simulink model "pd_path_sg"  (R2013b)
settings: Solver=ode45  StartTime=0.0  StopTime=10  RelTol=1e-3
undefined symbols (not defined in the file or in its folder): A, A2, B, C, D, EVAL, i, output_samp_bcoef, PCIN, reg_pk_lim, reg_plim, reg_scale, reg_sr_lim, reg_staclr, reg_txgain, THIS_DATE, W, X, Z
undefined symbols (not defined in the file): lut_address, lut_address_s5, reg_dltap
libraries: xbsIndex_r4 x3819, lut_ram_vhdl x32
(part 11 of 31)

== system pd_path_sg/output_sw_B/add_switch ==
  chi : Inport
  x : Inport  Port=2
  d : Inport  Port=3
  on0 : Inport  Port=4
  on1 : Inport  Port=5
  AddSub1 : xbsIndex_r4/AddSub  mode=Addition  use_carryin=off  use_carryout=off  en=off  latency=1  precision=User Defined  arith_type="Signed  (2's comp)"  n_bits=17  bin_pt=0  quantization=Truncate  overflow=Wrap  use_behavioral_HDL=off  hw_selection=Fabric  pipelined=off  dbl_ovrd=off  block_type=addsub
  AddSub2 : xbsIndex_r4/AddSub  mode=Addition  use_carryin=off  use_carryout=off  en=off  latency=1  precision=User Defined  arith_type="Signed  (2's comp)"  n_bits=17  bin_pt=0  quantization=Truncate  overflow=Wrap  use_behavioral_HDL=off  hw_selection=Fabric  pipelined=off  dbl_ovrd=off  block_type=addsub
  Constant : xbsIndex_r4/Constant  const=0  gui_display_data_type=Fixed-point  arith_type=Signed (2's comp)  n_bits=17  bin_pt=0  preci_type=Single  exp_width=8  frac_width=24  explicit_period=off  period=1  equ=P=C  opselect=C  inp2=PCIN>>17  opr=+  inp1=P  carry=CIN  dbl_ovrd=off  block_type=constant
  Constant1 : xbsIndex_r4/Constant  const=0  gui_display_data_type=Fixed-point  arith_type=Signed (2's comp)  n_bits=17  bin_pt=0  preci_type=Single  exp_width=8  frac_width=24  explicit_period=off  period=1  equ=P=C  opselect=C  inp2=PCIN>>17  opr=+  inp1=P  carry=CIN  dbl_ovrd=off  block_type=constant
  Delay : xbsIndex_r4/Delay  rst=off  infoeditControl=Selection of Reset will increase slice count due to use of real FFs and instead of SRLs  en=off  latency=delaytaps+1  reg_retiming=off  dbl_ovrd=off  block_type=delay
      settings: infoedit=Hardware notes: A delay line is a chain, each link of which is an SRL16 or SRL32 followed by a flip-flop.
  Delay1 : xbsIndex_r4/Delay  rst=off  infoeditControl=Selection of Reset will increase slice count due to use of real FFs and instead of SRLs  en=off  latency=delaytaps+1  reg_retiming=off  dbl_ovrd=off  block_type=delay
      settings: infoedit=Hardware notes: A delay line is a chain, each link of which is an SRL16 or SRL32 followed by a flip-flop.
  Delay2 : xbsIndex_r4/Delay  rst=off  infoeditControl=Selection of Reset will increase slice count due to use of real FFs and instead of SRLs  en=off  latency=delaytaps  reg_retiming=off  dbl_ovrd=off  block_type=delay
      settings: infoedit=Hardware notes: A delay line is a chain, each link of which is an SRL16 or SRL32 followed by a flip-flop.
  Delay3 : xbsIndex_r4/Delay  rst=off  infoeditControl=Selection of Reset will increase slice count due to use of real FFs and instead of SRLs  en=off  latency=delaytaps  reg_retiming=off  dbl_ovrd=off  block_type=delay
      settings: infoedit=Hardware notes: A delay line is a chain, each link of which is an SRL16 or SRL32 followed by a flip-flop.
  Delay4 : xbsIndex_r4/Delay  rst=off  infoeditControl=Selection of Reset will increase slice count due to use of real FFs and instead of SRLs  en=off  latency=delaytaps  reg_retiming=off  dbl_ovrd=off  block_type=delay
      settings: infoedit=Hardware notes: A delay line is a chain, each link of which is an SRL16 or SRL32 followed by a flip-flop.
  Delay5 : xbsIndex_r4/Delay  rst=off  infoeditControl=Selection of Reset will increase slice count due to use of real FFs and instead of SRLs  en=off  latency=2  reg_retiming=off  dbl_ovrd=off  block_type=delay
      settings: infoedit=Hardware notes: A delay line is a chain, each link of which is an SRL16 or SRL32 followed by a flip-flop.
  Demux1 : Demux  Outputs=2
  Demux2 : Demux  Outputs=2
  Mux : xbsIndex_r4/Mux  inputs=2  en=off  latency=1  precision=Full  arith_type=Unsigned  n_bits=16  bin_pt=14  quantization=Truncate  overflow=Wrap  dbl_ovrd=off  block_type=mux
  Mux1 : xbsIndex_r4/Mux  inputs=2  en=off  latency=0  precision=Full  arith_type=Unsigned  n_bits=16  bin_pt=14  quantization=Truncate  overflow=Wrap  dbl_ovrd=off  block_type=mux
  Mux2 : xbsIndex_r4/Mux  inputs=2  en=off  latency=1  precision=Full  arith_type=Unsigned  n_bits=16  bin_pt=14  quantization=Truncate  overflow=Wrap  dbl_ovrd=off  block_type=mux
  Mux3 : Mux  Inputs=2
  cho : Outport
  y : Outport  Port=2
  wires:
  Mux1/1 -> Mux/1, Mux2/1
  Delay5/1 -> cho/1
  Delay4/1 -> Mux1/1, Delay5/1
  Delay3/1 -> Mux2/3
  Delay2/1 -> Mux/3
  Delay1/1 -> AddSub2/1
  Delay/1 -> AddSub1/1
  Mux3/1 -> y/1
  AddSub2/1 -> Mux3/2
  AddSub1/1 -> Mux3/1
  Mux2/1 -> AddSub2/2
  Mux/1 -> AddSub1/2
  Demux2/2 -> Delay3/1
  Demux2/1 -> Delay2/1
  Constant1/1 -> Mux2/2
  Demux1/2 -> Delay1/1
  Demux1/1 -> Delay/1
  d/1 -> Demux2/1
  x/1 -> Demux1/1
  chi/1 -> Delay4/1
  on1/1 -> Mux1/3
  on0/1 -> Mux1/2
  Constant/1 -> Mux/2

== system pd_path_sg/output_sw_B/ch_split ==
  per : Inport
  chnsel : Inport  Port=2
  Bus Creator : BusCreator  Inputs=3
  Bus Creator1 : BusCreator  Inputs=3
  Bus Selector : BusSelector  OutputSignals=addr,din,we
  Constant : xbsIndex_r4/Constant  const=0  gui_display_data_type=Boolean  arith_type=Boolean  n_bits=16  bin_pt=14  preci_type=Single  exp_width=8  frac_width=24  explicit_period=off  period=1  equ=P=C  opselect=C  inp2=PCIN>>17  opr=+  inp1=P  carry=CIN  dbl_ovrd=off  block_type=constant
  Constant1 : xbsIndex_r4/Constant  const=0  gui_display_data_type=Boolean  arith_type=Boolean  n_bits=16  bin_pt=14  preci_type=Single  exp_width=8  frac_width=24  explicit_period=off  period=1  equ=P=C  opselect=C  inp2=PCIN>>17  opr=+  inp1=P  carry=CIN  dbl_ovrd=off  block_type=constant
  Mux : xbsIndex_r4/Mux  inputs=2  en=off  latency=0  precision=Full  arith_type=Unsigned  n_bits=16  bin_pt=14  quantization=Truncate  overflow=Wrap  dbl_ovrd=off  block_type=mux
  Mux1 : xbsIndex_r4/Mux  inputs=2  en=off  latency=0  precision=Full  arith_type=Unsigned  n_bits=16  bin_pt=14  quantization=Truncate  overflow=Wrap  dbl_ovrd=off  block_type=mux
  per0 : Outport
  per1 : Outport  Port=2
  wires:
  Bus Creator/1 -> per0/1
  Mux/1 -> Bus Creator/3  "we"
  Bus Creator1/1 -> per1/1
  Mux1/1 -> Bus Creator1/3  "we"
  Constant1/1 -> Mux1/2
  Bus Selector/3 -> Mux/2, Mux1/3  "<we>"
  Constant/1 -> Mux/3
  chnsel/1 -> Mux/1, Mux1/1
  Bus Selector/2 -> Bus Creator/2, Bus Creator1/2  "<din>"
  Bus Selector/1 -> Bus Creator/1, Bus Creator1/1  "<addr>"
  per/1 -> Bus Selector/1

== system pd_path_sg/output_sw_B/config_regs0 ==
  per : Inport
  rst : Inport  Port=2
  B0 : xbsIndex_r4/Slice  nbits=1  boolean_output=on  mode=Lower Bit Location + Width  bit1=0  base1=MSB of Input  bit0=0  base0=LSB of Input  dbl_ovrd=off  block_type=slice
  B1 : xbsIndex_r4/Slice  nbits=1  boolean_output=on  mode=Lower Bit Location + Width  bit1=0  base1=MSB of Input  bit0=1  base0=LSB of Input  dbl_ovrd=off  block_type=slice
  B2 : xbsIndex_r4/Slice  nbits=16  boolean_output=off  mode=Lower Bit Location + Width  bit1=0  base1=MSB of Input  bit0=0  base0=LSB of Input  dbl_ovrd=off  block_type=slice
  Bus Selector : BusSelector  OutputSignals=addr,din,we
  Slice : xbsIndex_r4/Slice  nbits=16  boolean_output=off  mode=Lower Bit Location + Width  bit1=0  base1=MSB of Input  bit0=0  base0=LSB of Input  dbl_ovrd=off  block_type=slice
  Slice1 : xbsIndex_r4/Slice  nbits=16  boolean_output=off  mode=Lower Bit Location + Width  bit1=0  base1=MSB of Input  bit0=0  base0=LSB of Input  dbl_ovrd=off  block_type=slice
  perbus_reg : Subsystem
  perbus_reg1 : Subsystem
  perbus_reg2 : Subsystem
  perbus_reg3 : Subsystem
  sr_lim : Outport
  pk_lim : Outport  Port=2
  alarm_clr : Outport  Port=3
  pd_on : Outport  Port=4
  tx_gain : Outport  Port=5
  wires:
  rst/1 -> perbus_reg3/4(rst), perbus_reg2/4(rst)
  B2/1 -> tx_gain/1
  perbus_reg3/1(q) -> B2/1
  B1/1 -> pd_on/1
  B0/1 -> alarm_clr/1
  perbus_reg2/1(q) -> B0/1, B1/1
  per/1 -> Bus Selector/1
  Bus Selector/1 -> perbus_reg/1(addr), perbus_reg1/1(addr), perbus_reg2/1(addr), perbus_reg3/1(addr)  "<addr>"
  Bus Selector/2 -> perbus_reg/2(din), perbus_reg2/2(din), perbus_reg3/2(din), perbus_reg1/2(din)  "<din>"
  Bus Selector/3 -> perbus_reg/3(we), perbus_reg1/3(we), perbus_reg2/3(we), perbus_reg3/3(we)  "<we>"
  perbus_reg/1(q) -> Slice/1
  perbus_reg1/1(q) -> Slice1/1
  Slice/1 -> sr_lim/1
  Slice1/1 -> pk_lim/1

== system pd_path_sg/output_sw_B/config_regs1 ==
  per : Inport
  rst : Inport  Port=2
  B0 : xbsIndex_r4/Slice  nbits=1  boolean_output=on  mode=Lower Bit Location + Width  bit1=0  base1=MSB of Input  bit0=0  base0=LSB of Input  dbl_ovrd=off  block_type=slice
  B1 : xbsIndex_r4/Slice  nbits=1  boolean_output=on  mode=Lower Bit Location + Width  bit1=0  base1=MSB of Input  bit0=1  base0=LSB of Input  dbl_ovrd=off  block_type=slice
  B2 : xbsIndex_r4/Slice  nbits=16  boolean_output=off  mode=Lower Bit Location + Width  bit1=0  base1=MSB of Input  bit0=0  base0=LSB of Input  dbl_ovrd=off  block_type=slice
  Bus Selector : BusSelector  OutputSignals=addr,din,we
  Slice : xbsIndex_r4/Slice  nbits=16  boolean_output=off  mode=Lower Bit Location + Width  bit1=0  base1=MSB of Input  bit0=0  base0=LSB of Input  dbl_ovrd=off  block_type=slice
  Slice1 : xbsIndex_r4/Slice  nbits=16  boolean_output=off  mode=Lower Bit Location + Width  bit1=0  base1=MSB of Input  bit0=0  base0=LSB of Input  dbl_ovrd=off  block_type=slice
  perbus_reg : Subsystem
  perbus_reg1 : Subsystem
  perbus_reg2 : Subsystem
  perbus_reg3 : Subsystem
  sr_lim : Outport
  pk_lim : Outport  Port=2
  alarm_clr : Outport  Port=3
  pd_on : Outport  Port=4
  tx_gain : Outport  Port=5
  wires:
  Slice1/1 -> pk_lim/1
  Slice/1 -> sr_lim/1
  perbus_reg1/1(q) -> Slice1/1
  perbus_reg/1(q) -> Slice/1
  Bus Selector/3 -> perbus_reg3/3(we), perbus_reg2/3(we), perbus_reg1/3(we), perbus_reg/3(we)  "<we>"
  Bus Selector/2 -> perbus_reg1/2(din), perbus_reg3/2(din), perbus_reg2/2(din), perbus_reg/2(din)  "<din>"
  Bus Selector/1 -> perbus_reg3/1(addr), perbus_reg2/1(addr), perbus_reg1/1(addr), perbus_reg/1(addr)  "<addr>"
  per/1 -> Bus Selector/1
  perbus_reg2/1(q) -> B1/1, B0/1
  B0/1 -> alarm_clr/1
  B1/1 -> pd_on/1
  perbus_reg3/1(q) -> B2/1
  B2/1 -> tx_gain/1
  rst/1 -> perbus_reg2/4(rst), perbus_reg3/4(rst)

== system pd_path_sg/output_sw_B/detect_i ==
  chi : Inport
  x : Inport  Port=2
  d : Inport  Port=3
  pk0 : Inport  Port=4
  pk1 : Inport  Port=5
  sr0 : Inport  Port=6
  sr1 : Inport  Port=7
  Absolute : xbsIndex_r4/Absolute  precision=User Defined  arith_type="Signed  (2's comp)"  n_bits=9  bin_pt=0  quantization=Truncate  overflow=Wrap  en=off  latency=0  dbl_ovrd=off  block_type=abs
  Absolute1 : xbsIndex_r4/Absolute  precision=User Defined  arith_type="Signed  (2's comp)"  n_bits=9  bin_pt=0  quantization=Truncate  overflow=Wrap  en=off  latency=0  dbl_ovrd=off  block_type=abs
  AddSub1 : xbsIndex_r4/AddSub  mode=Addition  use_carryin=off  use_carryout=off  en=off  latency=1  precision=User Defined  arith_type="Signed  (2's comp)"  n_bits=9  bin_pt=0  quantization=Truncate  overflow=Wrap  use_behavioral_HDL=off  hw_selection=Fabric  pipelined=off  dbl_ovrd=off  block_type=addsub
  AddSub2 : xbsIndex_r4/AddSub  mode=Subtraction  use_carryin=off  use_carryout=off  en=off  latency=1  precision=User Defined  arith_type="Signed  (2's comp)"  n_bits=9  bin_pt=0  quantization=Truncate  overflow=Wrap  use_behavioral_HDL=off  hw_selection=Fabric  pipelined=off  dbl_ovrd=off  block_type=addsub
  Delay : xbsIndex_r4/Delay  rst=off  infoeditControl=Selection of Reset will increase slice count due to use of real FFs and instead of SRLs  en=off  latency=2  reg_retiming=off  dbl_ovrd=off  block_type=delay
      settings: infoedit=Hardware notes: A delay line is a chain, each link of which is an SRL16 or SRL32 followed by a flip-flop.
  Delay1 : xbsIndex_r4/Delay  rst=off  infoeditControl=Selection of Reset will increase slice count due to use of real FFs and instead of SRLs  en=off  latency=2  reg_retiming=off  dbl_ovrd=off  block_type=delay
      settings: infoedit=Hardware notes: A delay line is a chain, each link of which is an SRL16 or SRL32 followed by a flip-flop.
  Mux : xbsIndex_r4/Mux  inputs=2  en=off  latency=1  precision=Full  arith_type=Unsigned  n_bits=16  bin_pt=14  quantization=Truncate  overflow=Wrap  dbl_ovrd=off  block_type=mux
  Mux1 : xbsIndex_r4/Mux  inputs=2  en=off  latency=1  precision=Full  arith_type=Unsigned  n_bits=16  bin_pt=14  quantization=Truncate  overflow=Wrap  dbl_ovrd=off  block_type=mux
  Relational : xbsIndex_r4/Relational  mode=a>b  op_type=Bool  en=off  latency=1  dbl_ovrd=off  block_type=relational
  Relational1 : xbsIndex_r4/Relational  mode=a>b  op_type=Bool  en=off  latency=1  dbl_ovrd=off  block_type=relational
  cut8bit : Subsystem
  cut8bit1 : Subsystem
  cut8bit2 : Subsystem
  cut8bit3 : Subsystem
  cut8bit4 : Subsystem
  cut8bit5 : Subsystem
  cho : Outport
  pk_alarm : Outport  Port=2
  sr_alarm : Outport  Port=3
  wires:
  cut8bit3/1(q) -> Mux/3
  cut8bit/1(q) -> AddSub1/1
  Delay1/1 -> cho/1
  Relational1/1 -> sr_alarm/1
  sr1/1 -> cut8bit5/1(d)
  sr0/1 -> cut8bit4/1(d)
  Mux1/1 -> Relational1/2
  AddSub2/1 -> Absolute1/1
  Absolute1/1 -> Relational1/1
  Delay/1 -> AddSub2/2
  cut8bit5/1(q) -> Mux1/3
  cut8bit4/1(q) -> Mux1/2
  chi/1 -> Mux1/1, Delay1/1, Mux/1
  cut8bit1/1(q) -> AddSub1/2, Delay/1, AddSub2/1
  Mux/1 -> Relational/2
  pk1/1 -> cut8bit3/1(d)
  cut8bit2/1(q) -> Mux/2
  Relational/1 -> pk_alarm/1
  Absolute/1 -> Relational/1
  AddSub1/1 -> Absolute/1
  pk0/1 -> cut8bit2/1(d)
  d/1 -> cut8bit1/1(d)
  x/1 -> cut8bit/1(d)

== system pd_path_sg/output_sw_B/detect_q ==
  chi : Inport
  x : Inport  Port=2
  d : Inport  Port=3
  pk0 : Inport  Port=4
  pk1 : Inport  Port=5
  sr0 : Inport  Port=6
  sr1 : Inport  Port=7
  Absolute : xbsIndex_r4/Absolute  precision=User Defined  arith_type="Signed  (2's comp)"  n_bits=9  bin_pt=0  quantization=Truncate  overflow=Wrap  en=off  latency=0  dbl_ovrd=off  block_type=abs
  Absolute1 : xbsIndex_r4/Absolute  precision=User Defined  arith_type="Signed  (2's comp)"  n_bits=9  bin_pt=0  quantization=Truncate  overflow=Wrap  en=off  latency=0  dbl_ovrd=off  block_type=abs
  AddSub1 : xbsIndex_r4/AddSub  mode=Addition  use_carryin=off  use_carryout=off  en=off  latency=1  precision=User Defined  arith_type="Signed  (2's comp)"  n_bits=9  bin_pt=0  quantization=Truncate  overflow=Wrap  use_behavioral_HDL=off  hw_selection=Fabric  pipelined=off  dbl_ovrd=off  block_type=addsub
  AddSub2 : xbsIndex_r4/AddSub  mode=Subtraction  use_carryin=off  use_carryout=off  en=off  latency=1  precision=User Defined  arith_type="Signed  (2's comp)"  n_bits=9  bin_pt=0  quantization=Truncate  overflow=Wrap  use_behavioral_HDL=off  hw_selection=Fabric  pipelined=off  dbl_ovrd=off  block_type=addsub
  Delay : xbsIndex_r4/Delay  rst=off  infoeditControl=Selection of Reset will increase slice count due to use of real FFs and instead of SRLs  en=off  latency=2  reg_retiming=off  dbl_ovrd=off  block_type=delay
      settings: infoedit=Hardware notes: A delay line is a chain, each link of which is an SRL16 or SRL32 followed by a flip-flop.
  Delay1 : xbsIndex_r4/Delay  rst=off  infoeditControl=Selection of Reset will increase slice count due to use of real FFs and instead of SRLs  en=off  latency=2  reg_retiming=off  dbl_ovrd=off  block_type=delay
      settings: infoedit=Hardware notes: A delay line is a chain, each link of which is an SRL16 or SRL32 followed by a flip-flop.
  Mux : xbsIndex_r4/Mux  inputs=2  en=off  latency=1  precision=Full  arith_type=Unsigned  n_bits=16  bin_pt=14  quantization=Truncate  overflow=Wrap  dbl_ovrd=off  block_type=mux
  Mux1 : xbsIndex_r4/Mux  inputs=2  en=off  latency=1  precision=Full  arith_type=Unsigned  n_bits=16  bin_pt=14  quantization=Truncate  overflow=Wrap  dbl_ovrd=off  block_type=mux
  Relational : xbsIndex_r4/Relational  mode=a>b  op_type=Bool  en=off  latency=1  dbl_ovrd=off  block_type=relational
  Relational1 : xbsIndex_r4/Relational  mode=a>b  op_type=Bool  en=off  latency=1  dbl_ovrd=off  block_type=relational
  cut8bit : Subsystem
  cut8bit1 : Subsystem
  cut8bit2 : Subsystem
  cut8bit3 : Subsystem
  cut8bit4 : Subsystem
  cut8bit5 : Subsystem
  cho : Outport
  pk_alarm : Outport  Port=2
  sr_alarm : Outport  Port=3
  wires:
  x/1 -> cut8bit/1(d)
  d/1 -> cut8bit1/1(d)
  pk0/1 -> cut8bit2/1(d)
  AddSub1/1 -> Absolute/1
  Absolute/1 -> Relational/1
  Relational/1 -> pk_alarm/1
  cut8bit2/1(q) -> Mux/2
  pk1/1 -> cut8bit3/1(d)
  Mux/1 -> Relational/2
  cut8bit1/1(q) -> AddSub2/1, Delay/1, AddSub1/2
  chi/1 -> Mux/1, Delay1/1, Mux1/1
  cut8bit4/1(q) -> Mux1/2
  cut8bit5/1(q) -> Mux1/3
  Delay/1 -> AddSub2/2
  Absolute1/1 -> Relational1/1
  AddSub2/1 -> Absolute1/1
  Mux1/1 -> Relational1/2
  sr0/1 -> cut8bit4/1(d)
  sr1/1 -> cut8bit5/1(d)
  Relational1/1 -> sr_alarm/1
  Delay1/1 -> cho/1
  cut8bit/1(q) -> AddSub1/1
  cut8bit3/1(q) -> Mux/3

== system pd_path_sg/output_sw_B/on_status ==
  chi : Inport
  pki_alarm : Inport  Port=2
  sri_alarm : Inport  Port=3
  pkq_alarm : Inport  Port=4
  srq_alarm : Inport  Port=5
  clr0 : Inport  Port=6
  clr1 : Inport  Port=7
  on0 : Inport  Port=8
  on1 : Inport  Port=9
  chnsel : Inport  Port=10
  Constant : xbsIndex_r4/Constant  const=0  gui_display_data_type=Boolean  arith_type=Boolean  n_bits=1  bin_pt=0  preci_type=Single  exp_width=8  frac_width=24  explicit_period=off  period=1  equ=P=C  opselect=C  inp2=PCIN>>17  opr=+  inp1=P  carry=CIN  dbl_ovrd=off  block_type=constant
  Constant{1..2,4..5} (4 alike) : xbsIndex_r4/Constant  const=1  gui_display_data_type=Boolean  arith_type=Boolean  n_bits=1  bin_pt=0  preci_type=Single  exp_width=8  frac_width=24  explicit_period=off  period=1  equ=P=C  opselect=C  inp2=PCIN>>17  opr=+  inp1=P  carry=CIN  dbl_ovrd=off  block_type=constant
  Constant3 : xbsIndex_r4/Constant  const=0  gui_display_data_type=Boolean  arith_type=Boolean  n_bits=1  bin_pt=0  preci_type=Single  exp_width=8  frac_width=24  explicit_period=off  period=1  equ=P=C  opselect=C  inp2=PCIN>>17  opr=+  inp1=P  carry=CIN  dbl_ovrd=off  block_type=constant
  Inverter : xbsIndex_r4/Inverter  en=off  latency=0  dbl_ovrd=off  block_type=inv
  Inverter1 : xbsIndex_r4/Inverter  en=off  latency=0  dbl_ovrd=off  block_type=inv
  Logical{,1..2,4,6..7} (6 alike) : xbsIndex_r4/Logical  logical_function=OR  inputs=2  en=off  latency=0  precision=Full  arith_type=Unsigned  n_bits=16  bin_pt=0  align_bp=on  dbl_ovrd=off  block_type=logical
  Logical3 : xbsIndex_r4/Logical  logical_function=AND  inputs=2  en=off  latency=0  precision=Full  arith_type=Unsigned  n_bits=16  bin_pt=0  align_bp=on  dbl_ovrd=off  block_type=logical
  Logical5 : xbsIndex_r4/Logical  logical_function=AND  inputs=2  en=off  latency=0  precision=Full  arith_type=Unsigned  n_bits=16  bin_pt=0  align_bp=on  dbl_ovrd=off  block_type=logical
  Mux{,1..3} (4 alike) : xbsIndex_r4/Mux  inputs=2  en=off  latency=0  precision=Full  arith_type=Unsigned  n_bits=16  bin_pt=14  quantization=Truncate  overflow=Wrap  dbl_ovrd=off  block_type=mux
  Mux4 : xbsIndex_r4/Mux  inputs=2  en=off  latency=1  precision=Full  arith_type=Unsigned  n_bits=16  bin_pt=14  quantization=Truncate  overflow=Wrap  dbl_ovrd=off  block_type=mux
  Mux5 : xbsIndex_r4/Mux  inputs=2  en=off  latency=1  precision=Full  arith_type=Unsigned  n_bits=16  bin_pt=14  quantization=Truncate  overflow=Wrap  dbl_ovrd=off  block_type=mux
  pk0 : xbsIndex_r4/Register  init=0  rst=on  en=on  dbl_ovrd=off  block_type=register
  pk1 : xbsIndex_r4/Register  init=0  rst=on  en=on  dbl_ovrd=off  block_type=register
  sr0 : xbsIndex_r4/Register  init=0  rst=on  en=on  dbl_ovrd=off  block_type=register
  sr1 : xbsIndex_r4/Register  init=0  rst=on  en=on  dbl_ovrd=off  block_type=register
  pk_status : Outport
  sr_status : Outport  Port=2
  sw0 : Outport  Port=3
  sw1 : Outport  Port=4
  wires:
  Logical/1 -> Mux/2
  on0/1 -> Logical3/1
  on1/1 -> Logical5/1
  Logical7/1 -> Mux3/3
  Logical6/1 -> Mux1/3
  clr1/1 -> pk1/2, sr1/2
  clr0/1 -> pk0/2, sr0/2
  Mux5/1 -> sr_status/1
  Mux4/1 -> pk_status/1
  chnsel/1 -> Mux4/1, Mux5/1
  chi/1 -> Mux/1, Mux1/1, Mux3/1, Mux2/1
  Logical5/1 -> sw1/1
  Logical3/1 -> sw0/1
  sr1/1 -> Logical4/2, Mux5/3
  pk1/1 -> Logical4/1, Mux4/3
  Inverter1/1 -> Logical5/2
  Logical4/1 -> Inverter1/1
  Inverter/1 -> Logical3/2
  Logical2/1 -> Inverter/1
  sr0/1 -> Logical2/2, Mux5/2
  pk0/1 -> Logical2/1, Mux4/2
  srq_alarm/1 -> Logical1/2, Logical7/2
  sri_alarm/1 -> Logical1/1, Logical7/1
  Mux3/1 -> sr1/3
  Constant5/1 -> sr1/1
  Constant4/1 -> sr0/1
  Mux2/1 -> sr0/3
  Constant3/1 -> Mux3/2, Mux2/3
  Logical1/1 -> Mux2/2
  Mux1/1 -> pk1/3
  Constant2/1 -> pk1/1
  Constant1/1 -> pk0/1
  Mux/1 -> pk0/3
  Constant/1 -> Mux/3, Mux1/2
  pkq_alarm/1 -> Logical/2, Logical6/2
  pki_alarm/1 -> Logical/1, Logical6/1

== system pd_path_sg/resamp_mod/LO1 ==
  rst : Inport
  Accumulator : xbsIndex_r4/Accumulator  operation=Add  n_bits=10  overflow=Wrap  scale=1  rst=on  hasbypass=off  infoeditControl=reset for floating point data type must be asserted for a minimum of 2 cycles  en=off  latency=1  msb_inp=100  msb=100  lsb=-100  use_behavioral_HDL=on  implementation=Fabric  dbl_ovrd=off  block_type=accum
  Constant : xbsIndex_r4/Constant  const=FTW  gui_display_data_type=Fixed-point  arith_type=Unsigned  n_bits=10  bin_pt=0  preci_type=Single  exp_width=8  frac_width=24  explicit_period=on  period=1  equ=P=C  opselect=C  inp2=PCIN>>17  opr=+  inp1=P  carry=CIN  dbl_ovrd=off  block_type=constant
  Convert : xbsIndex_r4/Convert  gui_display_data_type=Fixed-point  arith_type=Unsigned  n_bits=10  bin_pt=0  float_type=Single  exp_bits=8  fraction_bits=24  quantization=Truncate  overflow=Wrap  en=off  latency=0  pipeline=off  dbl_ovrd=off  block_type=convert
  Delay2 : xbsIndex_r4/Delay  rst=off  infoeditControl=Selection of Reset will increase slice count due to use of real FFs and instead of SRLs  en=off  latency=1  reg_retiming=off  dbl_ovrd=off  block_type=delay
      settings: infoedit=Hardware notes: A delay line is a chain, each link of which is an SRL16 or SRL32 followed by a flip-flop.
  Delay4 : xbsIndex_r4/Delay  rst=off  infoeditControl=Selection of Reset will increase slice count due to use of real FFs and instead of SRLs  en=off  latency=1  reg_retiming=off  dbl_ovrd=off  block_type=delay
      settings: infoedit=Hardware notes: A delay line is a chain, each link of which is an SRL16 or SRL32 followed by a flip-flop.
  ROM2 : xbsIndex_r4/ROM  depth=1024  initVector=LO_mod_coef  distributed_mem=Block RAM  rst=off  init_reg=0  en=off  latency=2  gui_display_data_type=Fixed-point  arith_type=Unsigned  n_bits=32  bin_pt=0  preci_type=Single  exp_width=8  frac_width=24  optimize=Area  use_rpm=on  dbl_ovrd=off  block_type=sprom
  Reinterpret1 : xbsIndex_r4/Reinterpret  force_arith_type=on  arith_type="Signed  (2's comp)"  force_bin_pt=on  bin_pt=14  block_type=reinterpret
  Reinterpret4 : xbsIndex_r4/Reinterpret  force_arith_type=on  arith_type="Signed  (2's comp)"  force_bin_pt=on  bin_pt=14  block_type=reinterpret
  Slice1 : xbsIndex_r4/Slice  nbits=16  boolean_output=off  mode=Lower Bit Location + Width  bit1=0  base1=MSB of Input  bit0=16  base0=LSB of Input  dbl_ovrd=off  block_type=slice
  Slice2 : xbsIndex_r4/Slice  nbits=16  boolean_output=off  mode=Lower Bit Location + Width  bit1=0  base1=MSB of Input  bit0=0  base0=LSB of Input  dbl_ovrd=off  block_type=slice
  sin : Outport
  cos : Outport  Port=2
  wires:
  rst/1 -> Accumulator/2
  Constant/1 -> Accumulator/1
  Accumulator/1 -> Convert/1
  Convert/1 -> Delay2/1
  Delay2/1 -> ROM2/1
  Slice2/1 -> Reinterpret4/1
  Slice1/1 -> Reinterpret1/1
  ROM2/1 -> Delay4/1
  Delay4/1 -> Slice1/1, Slice2/1
  Reinterpret4/1 -> cos/1
  Reinterpret1/1 -> sin/1

== system pd_path_sg/resamp_mod/mod0 ==
  Ai : Inport
  Aq : Inport  Port=2
  Bi : Inport  Port=3
  Bq : Inport  Port=4
  sin : Inport  Port=5
  cos : Inport  Port=6
  Delay{,1..3} (4 alike) : xbsIndex_r4/Delay  rst=off  infoeditControl=Selection of Reset will increase slice count due to use of real FFs and instead of SRLs  en=off  latency=1  reg_retiming=off  dbl_ovrd=off  block_type=delay
      settings: infoedit=Hardware notes: A delay line is a chain, each link of which is an SRL16 or SRL32 followed by a flip-flop.
  imag_modu : Subsystem
  real_modu : Subsystem
  Yi : Outport
  Yq : Outport  Port=2
  wires:
  sin/1 -> imag_modu/5(sin), real_modu/5(sin)
  Delay/1 -> imag_modu/1(Ai), real_modu/1(Ai)
  Delay1/1 -> imag_modu/2(Aq), real_modu/2(Aq)
  Delay2/1 -> imag_modu/3(Bi), real_modu/3(Bi)
  Delay3/1 -> imag_modu/4(Bq), real_modu/4(Bq)
  cos/1 -> imag_modu/6(cos), real_modu/6(cos)
  real_modu/1(out_real) -> Yi/1
  Ai/1 -> Delay/1
  Aq/1 -> Delay1/1
  Bi/1 -> Delay2/1
  Bq/1 -> Delay3/1
  imag_modu/1(out_imag) -> Yq/1

== system pd_path_sg/resamp_mod/mod1 ==
  Ai : Inport
  Aq : Inport  Port=2
  Bi : Inport  Port=3
  Bq : Inport  Port=4
  sin : Inport  Port=5
  cos : Inport  Port=6
  Delay{,1..3} (4 alike) : xbsIndex_r4/Delay  rst=off  infoeditControl=Selection of Reset will increase slice count due to use of real FFs and instead of SRLs  en=off  latency=1  reg_retiming=off  dbl_ovrd=off  block_type=delay
      settings: infoedit=Hardware notes: A delay line is a chain, each link of which is an SRL16 or SRL32 followed by a flip-flop.
  imag_modu : Subsystem
  real_modu : Subsystem
  Yi : Outport
  Yq : Outport  Port=2
  wires:
  imag_modu/1(out_imag) -> Yq/1
  Bq/1 -> Delay3/1
  Bi/1 -> Delay2/1
  Aq/1 -> Delay1/1
  Ai/1 -> Delay/1
  real_modu/1(out_real) -> Yi/1
  cos/1 -> real_modu/6(cos), imag_modu/6(cos)
  Delay3/1 -> real_modu/4(Bq), imag_modu/4(Bq)
  Delay2/1 -> real_modu/3(Bi), imag_modu/3(Bi)
  Delay1/1 -> real_modu/2(Aq), imag_modu/2(Aq)
  Delay/1 -> real_modu/1(Ai), imag_modu/1(Ai)
  sin/1 -> real_modu/5(sin), imag_modu/5(sin)

== system pd_path_sg/resamp_mod/output_samp_E2_p0 ==
  Ai : Inport
  chn : Inport  Port=2
  Delay1 : xbsIndex_r4/Delay  rst=off  infoeditControl=Selection of Reset will increase slice count due to use of real FFs and instead of SRLs  en=off  latency=1  reg_retiming=off  dbl_ovrd=off  block_type=delay
      settings: infoedit=Hardware notes: A delay line is a chain, each link of which is an SRL16 or SRL32 followed by a flip-flop.
  Mux : xbsIndex_r4/Mux  inputs=2  en=off  latency=1  precision=Full  arith_type=Unsigned  n_bits=16  bin_pt=14  quantization=Truncate  overflow=Wrap  dbl_ovrd=off  block_type=mux
  Mux1 : xbsIndex_r4/Mux  inputs=2  en=off  latency=1  precision=Full  arith_type=Unsigned  n_bits=16  bin_pt=14  quantization=Truncate  overflow=Wrap  dbl_ovrd=off  block_type=mux
  up_sampi : Subsystem
  Ai0 : Outport
  Ai1 : Outport  Port=2
  wires:
  Delay1/1 -> Ai0/1
  Mux1/1 -> Ai1/1
  Mux/1 -> Delay1/1
  chn/1 -> Mux/1, Mux1/1
  up_sampi/2(Out1) -> Mux/3, Mux1/2
  up_sampi/1(Out0) -> Mux/2, Mux1/3
  Ai/1 -> up_sampi/1(In1)

== system pd_path_sg/resamp_mod/output_samp_E2_p1 ==
  Ai : Inport
  chn : Inport  Port=2
  Delay1 : xbsIndex_r4/Delay  rst=off  infoeditControl=Selection of Reset will increase slice count due to use of real FFs and instead of SRLs  en=off  latency=1  reg_retiming=off  dbl_ovrd=off  block_type=delay
      settings: infoedit=Hardware notes: A delay line is a chain, each link of which is an SRL16 or SRL32 followed by a flip-flop.
  Mux : xbsIndex_r4/Mux  inputs=2  en=off  latency=1  precision=Full  arith_type=Unsigned  n_bits=16  bin_pt=14  quantization=Truncate  overflow=Wrap  dbl_ovrd=off  block_type=mux
  Mux1 : xbsIndex_r4/Mux  inputs=2  en=off  latency=1  precision=Full  arith_type=Unsigned  n_bits=16  bin_pt=14  quantization=Truncate  overflow=Wrap  dbl_ovrd=off  block_type=mux
  up_sampi : Subsystem
  Ai0 : Outport
  Ai1 : Outport  Port=2
  wires:
  Ai/1 -> up_sampi/1(In1)
  up_sampi/1(Out0) -> Mux1/3, Mux/2
  up_sampi/2(Out1) -> Mux1/2, Mux/3
  chn/1 -> Mux1/1, Mux/1
  Mux/1 -> Delay1/1
  Mux1/1 -> Ai1/1
  Delay1/1 -> Ai0/1

== system pd_path_sg/resamp_mod/output_samp_E2_p2 ==
  Ai : Inport
  chn : Inport  Port=2
  Delay1 : xbsIndex_r4/Delay  rst=off  infoeditControl=Selection of Reset will increase slice count due to use of real FFs and instead of SRLs  en=off  latency=1  reg_retiming=off  dbl_ovrd=off  block_type=delay
      settings: infoedit=Hardware notes: A delay line is a chain, each link of which is an SRL16 or SRL32 followed by a flip-flop.
  Mux : xbsIndex_r4/Mux  inputs=2  en=off  latency=1  precision=Full  arith_type=Unsigned  n_bits=16  bin_pt=14  quantization=Truncate  overflow=Wrap  dbl_ovrd=off  block_type=mux
  Mux1 : xbsIndex_r4/Mux  inputs=2  en=off  latency=1  precision=Full  arith_type=Unsigned  n_bits=16  bin_pt=14  quantization=Truncate  overflow=Wrap  dbl_ovrd=off  block_type=mux
  up_sampi : Subsystem
  Ai0 : Outport
  Ai1 : Outport  Port=2
  wires:
  Delay1/1 -> Ai0/1
  Mux1/1 -> Ai1/1
  Mux/1 -> Delay1/1
  chn/1 -> Mux/1, Mux1/1
  up_sampi/2(Out1) -> Mux/3, Mux1/2
  up_sampi/1(Out0) -> Mux/2, Mux1/3
  Ai/1 -> up_sampi/1(In1)

== system pd_path_sg/resamp_mod/output_samp_E2_p3 ==
  Ai : Inport
  chn : Inport  Port=2
  Delay1 : xbsIndex_r4/Delay  rst=off  infoeditControl=Selection of Reset will increase slice count due to use of real FFs and instead of SRLs  en=off  latency=1  reg_retiming=off  dbl_ovrd=off  block_type=delay
      settings: infoedit=Hardware notes: A delay line is a chain, each link of which is an SRL16 or SRL32 followed by a flip-flop.
  Mux : xbsIndex_r4/Mux  inputs=2  en=off  latency=1  precision=Full  arith_type=Unsigned  n_bits=16  bin_pt=14  quantization=Truncate  overflow=Wrap  dbl_ovrd=off  block_type=mux
  Mux1 : xbsIndex_r4/Mux  inputs=2  en=off  latency=1  precision=Full  arith_type=Unsigned  n_bits=16  bin_pt=14  quantization=Truncate  overflow=Wrap  dbl_ovrd=off  block_type=mux
  up_sampi : Subsystem
  Ai0 : Outport
  Ai1 : Outport  Port=2
  wires:
  Ai/1 -> up_sampi/1(In1)
  up_sampi/1(Out0) -> Mux1/3, Mux/2
  up_sampi/2(Out1) -> Mux1/2, Mux/3
  chn/1 -> Mux1/1, Mux/1
  Mux/1 -> Delay1/1
  Mux1/1 -> Ai1/1
  Delay1/1 -> Ai0/1

== system pd_path_sg/A_dispatch/config_regs/perbus_reg ==
  addr : Inport
  din : Inport  Port=2
  we : Inport  Port=3
  Logical1 : xbsIndex_r4/Logical  logical_function=AND  inputs=2  en=off  latency=0  precision=Full  arith_type=Unsigned  n_bits=16  bin_pt=0  align_bp=on  dbl_ovrd=off  block_type=logical
  REG_ADDR : xbsIndex_r4/Constant  const=reg_addr  gui_display_data_type=Fixed-point  arith_type=Unsigned  n_bits=12  bin_pt=0  preci_type=Single  exp_width=8  frac_width=24  explicit_period=off  period=1  equ=P=C  opselect=C  inp2=PCIN>>17  opr=+  inp1=P  carry=CIN  dbl_ovrd=off  block_type=constant
  Register : xbsIndex_r4/Register  init=0  rst=off  en=on  dbl_ovrd=off  block_type=register
  Relational2 : xbsIndex_r4/Relational  mode=a=b  op_type=Bool  en=off  latency=0  dbl_ovrd=off  block_type=relational
  q : Outport
  wires:
  REG_ADDR/1 -> Relational2/2
  Relational2/1 -> Logical1/2
  Logical1/1 -> Register/2
  addr/1 -> Relational2/1
  we/1 -> Logical1/1
  din/1 -> Register/1
  Register/1 -> q/1

== system pd_path_sg/A_dispatch/config_regs/perbus_reg1 ==
  addr : Inport
  din : Inport  Port=2
  we : Inport  Port=3
  Logical1 : xbsIndex_r4/Logical  logical_function=AND  inputs=2  en=off  latency=0  precision=Full  arith_type=Unsigned  n_bits=16  bin_pt=0  align_bp=on  dbl_ovrd=off  block_type=logical
  REG_ADDR : xbsIndex_r4/Constant  const=reg_addr  gui_display_data_type=Fixed-point  arith_type=Unsigned  n_bits=12  bin_pt=0  preci_type=Single  exp_width=8  frac_width=24  explicit_period=off  period=1  equ=P=C  opselect=C  inp2=PCIN>>17  opr=+  inp1=P  carry=CIN  dbl_ovrd=off  block_type=constant
  Register : xbsIndex_r4/Register  init=0  rst=off  en=on  dbl_ovrd=off  block_type=register
  Relational2 : xbsIndex_r4/Relational  mode=a=b  op_type=Bool  en=off  latency=0  dbl_ovrd=off  block_type=relational
  q : Outport
  wires:
  Register/1 -> q/1
  din/1 -> Register/1
  we/1 -> Logical1/1
  addr/1 -> Relational2/1
  Logical1/1 -> Register/2
  Relational2/1 -> Logical1/2
  REG_ADDR/1 -> Relational2/2

== system pd_path_sg/A_dispatch/config_regs/perbus_reg2 ==
  addr : Inport
  din : Inport  Port=2
  we : Inport  Port=3
  Logical1 : xbsIndex_r4/Logical  logical_function=AND  inputs=2  en=off  latency=0  precision=Full  arith_type=Unsigned  n_bits=16  bin_pt=0  align_bp=on  dbl_ovrd=off  block_type=logical
  REG_ADDR : xbsIndex_r4/Constant  const=reg_addr  gui_display_data_type=Fixed-point  arith_type=Unsigned  n_bits=12  bin_pt=0  preci_type=Single  exp_width=8  frac_width=24  explicit_period=off  period=1  equ=P=C  opselect=C  inp2=PCIN>>17  opr=+  inp1=P  carry=CIN  dbl_ovrd=off  block_type=constant
  Register : xbsIndex_r4/Register  init=0  rst=off  en=on  dbl_ovrd=off  block_type=register
  Relational2 : xbsIndex_r4/Relational  mode=a=b  op_type=Bool  en=off  latency=0  dbl_ovrd=off  block_type=relational
  q : Outport
  wires:
  REG_ADDR/1 -> Relational2/2
  Relational2/1 -> Logical1/2
  Logical1/1 -> Register/2
  addr/1 -> Relational2/1
  we/1 -> Logical1/1
  din/1 -> Register/1
  Register/1 -> q/1

== system pd_path_sg/A_dispatch/config_regs/perbus_reg3 ==
  addr : Inport
  din : Inport  Port=2
  we : Inport  Port=3
  Logical1 : xbsIndex_r4/Logical  logical_function=AND  inputs=2  en=off  latency=0  precision=Full  arith_type=Unsigned  n_bits=16  bin_pt=0  align_bp=on  dbl_ovrd=off  block_type=logical
  REG_ADDR : xbsIndex_r4/Constant  const=reg_addr  gui_display_data_type=Fixed-point  arith_type=Unsigned  n_bits=12  bin_pt=0  preci_type=Single  exp_width=8  frac_width=24  explicit_period=off  period=1  equ=P=C  opselect=C  inp2=PCIN>>17  opr=+  inp1=P  carry=CIN  dbl_ovrd=off  block_type=constant
  Register : xbsIndex_r4/Register  init=0  rst=off  en=on  dbl_ovrd=off  block_type=register
  Relational2 : xbsIndex_r4/Relational  mode=a=b  op_type=Bool  en=off  latency=0  dbl_ovrd=off  block_type=relational
  q : Outport
  wires:
  Register/1 -> q/1
  din/1 -> Register/1
  we/1 -> Logical1/1
  addr/1 -> Relational2/1
  Logical1/1 -> Register/2
  Relational2/1 -> Logical1/2
  REG_ADDR/1 -> Relational2/2

== system pd_path_sg/A_dispatch/config_regs/perbus_reg4 ==
  addr : Inport
  din : Inport  Port=2
  we : Inport  Port=3
  Logical1 : xbsIndex_r4/Logical  logical_function=AND  inputs=2  en=off  latency=0  precision=Full  arith_type=Unsigned  n_bits=16  bin_pt=0  align_bp=on  dbl_ovrd=off  block_type=logical
  REG_ADDR : xbsIndex_r4/Constant  const=reg_addr  gui_display_data_type=Fixed-point  arith_type=Unsigned  n_bits=12  bin_pt=0  preci_type=Single  exp_width=8  frac_width=24  explicit_period=off  period=1  equ=P=C  opselect=C  inp2=PCIN>>17  opr=+  inp1=P  carry=CIN  dbl_ovrd=off  block_type=constant
  Register : xbsIndex_r4/Register  init=0  rst=off  en=on  dbl_ovrd=off  block_type=register
  Relational2 : xbsIndex_r4/Relational  mode=a=b  op_type=Bool  en=off  latency=0  dbl_ovrd=off  block_type=relational
  q : Outport
  wires:
  REG_ADDR/1 -> Relational2/2
  Relational2/1 -> Logical1/2
  Logical1/1 -> Register/2
  addr/1 -> Relational2/1
  we/1 -> Logical1/1
  din/1 -> Register/1
  Register/1 -> q/1

== system pd_path_sg/A_dispatch/config_regs/perbus_reg5 ==
  addr : Inport
  din : Inport  Port=2
  we : Inport  Port=3
  Logical1 : xbsIndex_r4/Logical  logical_function=AND  inputs=2  en=off  latency=0  precision=Full  arith_type=Unsigned  n_bits=16  bin_pt=0  align_bp=on  dbl_ovrd=off  block_type=logical
  REG_ADDR : xbsIndex_r4/Constant  const=reg_addr  gui_display_data_type=Fixed-point  arith_type=Unsigned  n_bits=12  bin_pt=0  preci_type=Single  exp_width=8  frac_width=24  explicit_period=off  period=1  equ=P=C  opselect=C  inp2=PCIN>>17  opr=+  inp1=P  carry=CIN  dbl_ovrd=off  block_type=constant
  Register : xbsIndex_r4/Register  init=0  rst=off  en=on  dbl_ovrd=off  block_type=register
  Relational2 : xbsIndex_r4/Relational  mode=a=b  op_type=Bool  en=off  latency=0  dbl_ovrd=off  block_type=relational
  q : Outport
  wires:
  Register/1 -> q/1
  din/1 -> Register/1
  we/1 -> Logical1/1
  addr/1 -> Relational2/1
  Logical1/1 -> Register/2
  Relational2/1 -> Logical1/2
  REG_ADDR/1 -> Relational2/2

== system pd_path_sg/A_dispatch/config_regs/perbus_reg6 ==
  addr : Inport
  din : Inport  Port=2
  we : Inport  Port=3
  Logical1 : xbsIndex_r4/Logical  logical_function=AND  inputs=2  en=off  latency=0  precision=Full  arith_type=Unsigned  n_bits=16  bin_pt=0  align_bp=on  dbl_ovrd=off  block_type=logical
  REG_ADDR : xbsIndex_r4/Constant  const=reg_addr  gui_display_data_type=Fixed-point  arith_type=Unsigned  n_bits=12  bin_pt=0  preci_type=Single  exp_width=8  frac_width=24  explicit_period=off  period=1  equ=P=C  opselect=C  inp2=PCIN>>17  opr=+  inp1=P  carry=CIN  dbl_ovrd=off  block_type=constant
  Register : xbsIndex_r4/Register  init=0  rst=off  en=on  dbl_ovrd=off  block_type=register
  Relational2 : xbsIndex_r4/Relational  mode=a=b  op_type=Bool  en=off  latency=0  dbl_ovrd=off  block_type=relational
  q : Outport
  wires:
  REG_ADDR/1 -> Relational2/2
  Relational2/1 -> Logical1/2
  Logical1/1 -> Register/2
  addr/1 -> Relational2/1
  we/1 -> Logical1/1
  din/1 -> Register/1
  Register/1 -> q/1

== system pd_path_sg/A_lut_store/one_lut0/B ==
  d : Inport
  Delay : xbsIndex_r4/Delay  rst=off  infoeditControl=Selection of Reset will increase slice count due to use of real FFs and instead of SRLs  en=off  latency=1  reg_retiming=off  dbl_ovrd=off  block_type=delay
      settings: infoedit=Hardware notes: A delay line is a chain, each link of which is an SRL16 or SRL32 followed by a flip-flop.
  Slice : xbsIndex_r4/Slice  nbits=3  boolean_output=off  mode=Lower Bit Location + Width  bit1=0  base1=MSB of Input  bit0=1  base0=LSB of Input  dbl_ovrd=off  block_type=slice
  q : Outport
  wires:
  d/1 -> Delay/1
  Slice/1 -> q/1
  Delay/1 -> Slice/1

== system pd_path_sg/A_lut_store/one_lut0/Bf ==
  iaddr : Inport
  delta : Inport  Port=2
  AddSub : xbsIndex_r4/AddSub  mode=Subtraction  use_carryin=off  use_carryout=off  en=off  latency=0  precision=Full  arith_type=Unsigned  n_bits=16  bin_pt=14  quantization=Truncate  overflow=Wrap  use_behavioral_HDL=off  hw_selection=Fabric  pipelined=off  dbl_ovrd=off  block_type=addsub
  Constant : xbsIndex_r4/Constant  const=1.0  gui_display_data_type=Fixed-point  arith_type=Unsigned  n_bits=6  bin_pt=5  preci_type=Single  exp_width=8  frac_width=24  explicit_period=off  period=1  equ=P=C  opselect=C  inp2=PCIN>>17  opr=+  inp1=P  carry=CIN  dbl_ovrd=off  block_type=constant
  Convert : xbsIndex_r4/Convert  gui_display_data_type=Fixed-point  arith_type=Unsigned  n_bits=6  bin_pt=6  float_type=Single  exp_bits=8  fraction_bits=24  quantization=Truncate  overflow=Wrap  en=off  latency=0  pipeline=off  dbl_ovrd=off  block_type=convert
  Mux : xbsIndex_r4/Mux  inputs=2  en=off  latency=1  precision=Full  arith_type=Unsigned  n_bits=16  bin_pt=14  quantization=Truncate  overflow=Wrap  dbl_ovrd=off  block_type=mux
  Reinterpret : xbsIndex_r4/Reinterpret  force_arith_type=on  arith_type=Unsigned  force_bin_pt=on  bin_pt=6  block_type=reinterpret
  Slice : xbsIndex_r4/Slice  nbits=1  boolean_output=off  mode=Lower Bit Location + Width  bit1=0  base1=MSB of Input  bit0=0  base0=LSB of Input  dbl_ovrd=off  block_type=slice
  q : Outport
  wires:
  iaddr/1 -> Slice/1
  AddSub/1 -> Mux/3
  Mux/1 -> q/1
  Constant/1 -> AddSub/1
  delta/1 -> Reinterpret/1
  Slice/1 -> Mux/1
  Reinterpret/1 -> Convert/1
  Convert/1 -> AddSub/2, Mux/2

== system pd_path_sg/A_lut_store/one_lut0/Bp1 ==
  d : Inport
  AddSub : xbsIndex_r4/AddSub  mode=Addition  use_carryin=off  use_carryout=off  en=off  latency=1  precision=Full  arith_type=Unsigned  n_bits=16  bin_pt=14  quantization=Truncate  overflow=Wrap  use_behavioral_HDL=off  hw_selection=Fabric  pipelined=off  dbl_ovrd=off  block_type=addsub
  Constant : xbsIndex_r4/Constant  const=1.0  gui_display_data_type=Fixed-point  arith_type=Unsigned  n_bits=4  bin_pt=0  preci_type=Single  exp_width=8  frac_width=24  explicit_period=off  period=1  equ=P=C  opselect=C  inp2=PCIN>>17  opr=+  inp1=P  carry=CIN  dbl_ovrd=off  block_type=constant
  Slice : xbsIndex_r4/Slice  nbits=3  boolean_output=off  mode=Lower Bit Location + Width  bit1=0  base1=MSB of Input  bit0=1  base0=LSB of Input  dbl_ovrd=off  block_type=slice
  q : Outport
  wires:
  d/1 -> AddSub/1
  Constant/1 -> AddSub/2
  AddSub/1 -> Slice/1
  Slice/1 -> q/1

== system pd_path_sg/A_lut_store/one_lut0/addr_gen ==
  chn : Inport
  active0 : Inport  Port=2
  active1 : Inport  Port=3
  addr0 : Inport  Port=4
  addr1 : Inport  Port=5
  Concat : xbsIndex_r4/Concat  num_inputs=3  dbl_ovrd=off  block_type=concat
  Concat1 : xbsIndex_r4/Concat  num_inputs=3  dbl_ovrd=off  block_type=concat
  Delay : xbsIndex_r4/Delay  rst=off  infoeditControl=Selection of Reset will increase slice count due to use of real FFs and instead of SRLs  en=off  latency=1  reg_retiming=off  dbl_ovrd=off  block_type=delay
      settings: infoedit=Hardware notes: A delay line is a chain, each link of which is an SRL16 or SRL32 followed by a flip-flop.
  Delay1 : xbsIndex_r4/Delay  rst=off  infoeditControl=Selection of Reset will increase slice count due to use of real FFs and instead of SRLs  en=off  latency=1  reg_retiming=off  dbl_ovrd=off  block_type=delay
      settings: infoedit=Hardware notes: A delay line is a chain, each link of which is an SRL16 or SRL32 followed by a flip-flop.
  Mux : xbsIndex_r4/Mux  inputs=2  en=off  latency=1  precision=Full  arith_type=Unsigned  n_bits=16  bin_pt=14  quantization=Truncate  overflow=Wrap  dbl_ovrd=off  block_type=mux
  Mux1 : xbsIndex_r4/Mux  inputs=2  en=off  latency=1  precision=Full  arith_type=Unsigned  n_bits=16  bin_pt=14  quantization=Truncate  overflow=Wrap  dbl_ovrd=off  block_type=mux
  rd_addr0 : Outport
  rd_addr1 : Outport  Port=2
  wires:
  addr1/1 -> Concat1/3
  Concat1/1 -> rd_addr1/1
  Concat/1 -> rd_addr0/1  "rd_addr"
  addr0/1 -> Concat/3
  Delay/1 -> Concat/1
  Mux/1 -> Concat/2
  chn/1 -> Mux1/1, Delay1/1, Mux/1, Delay/1
  active0/1 -> Mux1/2, Mux/2
  active1/1 -> Mux1/3, Mux/3
  Mux1/1 -> Concat1/2
  Delay1/1 -> Concat1/1
